simulink model "sampleModel1884_2_sub"  (R2023a)
settings: Solver=VariableStepAuto  StartTime=0.0  StopTime=10.0  RelTol=1e-3
libraries: hdlsllib x6, simulink x2
settings Model: Creator=user1  LastModifiedBy=user1

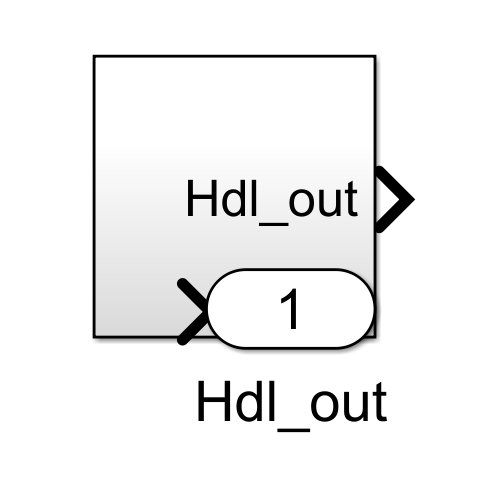
[thumbnail: Simulink's stored preview of the top-level diagram]
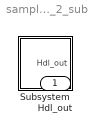
== system sampleModel1884_2_sub ==
  Subsystem : Subsystem
  Hdl_out : Outport  OutDataTypeStr=uint8

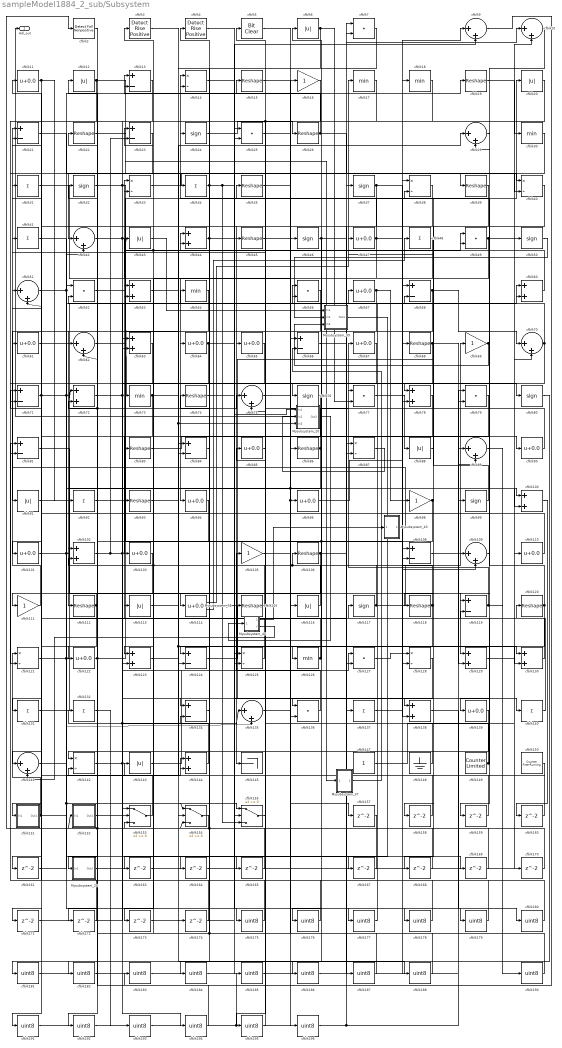
== system sampleModel1884_2_sub/Subsystem ==
  Mysubsystem_20 : Subsystem  TreatAsAtomicUnit=on  RTWFcnName=Mysubsystem_20
      settings: RTWFcnNameOpts=User specified  RTWFileNameOpts=Use function name
  Mysubsystem_28 : Subsystem  TreatAsAtomicUnit=on  RTWFcnName=Mysubsystem_28
      settings: RTWFcnNameOpts=User specified  RTWFileNameOpts=Use function name
  Mysubsystem_37 : Subsystem  TreatAsAtomicUnit=on  RTWFcnName=Mysubsystem_37
      settings: RTWFcnNameOpts=User specified  RTWFileNameOpts=Use function name
  Mysubsystem_38 : Subsystem  TreatAsAtomicUnit=on  RTWFcnName=Mysubsystem_38
      settings: RTWFcnNameOpts=User specified  RTWFileNameOpts=Use function name
  Mysubsystem_39 : Subsystem  TreatAsAtomicUnit=on  RTWFcnName=Mysubsystem_39
      settings: RTWFcnNameOpts=User specified  RTWFileNameOpts=Use function name
  Mysubsystem_40 : Subsystem  TreatAsAtomicUnit=on  RTWFcnName=Mysubsystem_40
      settings: RTWFcnNameOpts=User specified  RTWFileNameOpts=Use function name
  Mysubsystem_43 : Subsystem  TreatAsAtomicUnit=on  RTWFcnName=Mysubsystem_43
      settings: RTWFcnNameOpts=User specified  RTWFileNameOpts=Use function name
  cfblk{9..10,29,42,51,62,70,75,89,109,135,141} (12 alike) : Sum  Inputs=|++  OutDataTypeStr=uint8
  cfblk{44,53,60,63,72,78,100,102,123,129..130,138,144} (13 alike) : Sum  OutDataTypeStr=uint8
  cfblk{11,47,57,61,64..65,67,85,90,94,96,101,103,110,114,122,139} (17 alike) : Bias  Bias=0.0  SaturateOnIntegerOverflow=off
  cfblk{16,69,98,105,111} (5 alike) : Gain  OutDataTypeStr=uint8
  cfblk{15,19,22,26,35,39,45,68,74,83,86,93,106,112,115,118,120} (17 alike) : Reshape
  cfblk{13,21,23,58,66,71,81,84,108,119,124,134} (12 alike) : Sum  Inputs=+-  OutDataTypeStr=uint8
  cfblk{6,12,20,43,88,91,113,116,143} (9 alike) : Abs  OutDataTypeStr=uint8  SaturateOnIntegerOverflow=off
  cfblk{24,32,37,46,50,76,80,99,117} (9 alike) : Signum
  cfblk{14,33,38,40,87,121,125,128,142} (9 alike) : Product  Inputs=*/  OutDataTypeStr=uint8  RndMeth=Zero  SaturateOnIntegerOverflow=on
  cfblk{17..18,30,54,73,126} (6 alike) : MinMax  OutDataTypeStr=uint8
  cfblk{7,25,49,52,56,77,79,127,136} (9 alike) : DotProduct  OutDataTypeStr=uint8
  cfblk{31,34,41,48,92,131..132,137,140} (9 alike) : Sum  Inputs=+  OutDataTypeStr=uint8
  cfblk145 : Terminator
  cfblk147 : Constant  OutDataTypeStr=uint8  SampleTime=-1
  cfblk148 : Ground
  cfblk149 : hdlsllib/Sources/Counter Limited  uplimit=7  tsamp=-1
  cfblk150 : hdlsllib/Sources/Counter Free-Running  NumBits=16  tsamp=-1
  cfblk151 : Subsystem
      settings: LibrarySourceBlock=|
      | hdlsllib/Ports &
      | Subsystems/Subsystem
  cfblk152 : Subsystem
      settings: LibrarySourceBlock=|
      | hdlsllib/Ports &
      | Subsystems/Subsystem
  cfblk153 : Switch  OutDataTypeStr=uint8  SaturateOnIntegerOverflow=off  InputSameDT=off
  cfblk154 : Switch  OutDataTypeStr=uint8  SaturateOnIntegerOverflow=off  InputSameDT=off
  cfblk155 : Switch  OutDataTypeStr=uint8  SaturateOnIntegerOverflow=off  InputSameDT=off
  cfblk{157..161,163..165,167..174} (16 alike) : Delay  SampleTime=1
  cfblk{175..188,190..196} (21 alike) : DataTypeConversion  OutDataTypeStr=uint8  SaturateOnIntegerOverflow=off  RndMeth=Floor
  cfblk2 : hdlsllib/Logic and Bit Operations/Detect Fall Nonpositive  vinit=0  OutDataTypeStr=uint8
  cfblk3 : hdlsllib/Logic and Bit Operations/Detect Rise Positive  vinit=0  OutDataTypeStr=uint8
  cfblk4 : hdlsllib/Logic and Bit Operations/Detect Rise Positive  vinit=0  OutDataTypeStr=uint8
  cfblk5 : simulink/Logic and Bit Operations/Bit Clear  iBit=0
      settings: LibrarySourceBlock=|
      | hdlsllib/Logic and Bit
      | Operations/Bit Clear
  Hdl_out : Outport  OutDataTypeStr=uint8
  wires:
  cfblk73/1 -> cfblk188/1, cfblk83/1
  cfblk29/1 -> cfblk139/1
  cfblk139/1 -> cfblk142/1
  cfblk124/1 -> cfblk17/1
  cfblk122/1 -> cfblk62/2, cfblk49/1
  cfblk111/1 -> cfblk21/1
  cfblk98/1 -> cfblk168/1, cfblk186/1, cfblk154/2
  cfblk56/1 -> cfblk91/1
  cfblk69/1 -> cfblk119/1, Mysubsystem_39/3(In3)
  cfblk49/1 -> cfblk118/1, cfblk50/1
  cfblk114/1 -> cfblk140/1
  cfblk24/1 -> cfblk26/1
  cfblk131/1 -> cfblk16/1
  cfblk112/1 -> cfblk141/1, cfblk111/1
  cfblk118/1 -> cfblk134/1, cfblk53/1, cfblk106/1
  cfblk150/1 -> cfblk142/2
  cfblk83/1 -> cfblk90/1
  cfblk39/1 -> cfblk145/1
  cfblk151/1(Out1) -> cfblk121/1, cfblk154/1, cfblk144/1
  cfblk54/1 -> cfblk112/1
  cfblk88/1 -> cfblk117/1
  cfblk53/1 -> cfblk167/1, cfblk129/2
  cfblk47/1 -> cfblk9/1, cfblk123/1, cfblk14/1
  cfblk48/1 -> cfblk94/1
  cfblk63/1 -> cfblk81/2
  cfblk31/1 -> cfblk86/1
  cfblk16/1 -> cfblk65/1, cfblk121/2
  cfblk119/1 -> cfblk170/1, cfblk67/1
  cfblk108/1 -> cfblk69/1
  cfblk17/1 -> cfblk114/1
  cfblk93/1 -> cfblk29/1, Mysubsystem_20/3(In3)
  cfblk79/1 -> cfblk138/1
  cfblk40/1 -> cfblk78/1
  cfblk121/1 -> cfblk60/2, cfblk87/1
  cfblk144/1 -> cfblk12/1
  cfblk136/1 -> cfblk105/1
  cfblk26/1 -> cfblk40/2, cfblk15/1
  cfblk89/1 -> cfblk190/1
  cfblk127/1 -> cfblk128/1
  cfblk94/1 -> cfblk122/1
  cfblk71/1 -> cfblk51/2, cfblk13/2, cfblk60/1
  cfblk130/1 -> cfblk33/1
  cfblk148/1 -> cfblk41/1
  cfblk57/1 -> cfblk98/1, cfblk115/1
  cfblk76/1 -> cfblk103/1
  cfblk81/1 -> cfblk125/1
  cfblk92/1 -> cfblk24/1
  cfblk137/1 -> cfblk109/1
  cfblk152/1(Out1) -> cfblk135/1, cfblk127/1
  cfblk10/1 -> cfblk29/2
  cfblk14/1 -> cfblk45/1
  cfblk58/1 -> cfblk93/1, cfblk70/1
  cfblk115/1 -> cfblk53/2, cfblk22/1
  cfblk126/1 -> cfblk6/1, cfblk31/1
  cfblk32/1 -> cfblk155/1, cfblk108/2
  cfblk102/1 -> cfblk23/2, cfblk155/2, cfblk58/2
  cfblk128/1 -> cfblk153/2
  cfblk155/1 -> cfblk85/1
  cfblk62/1 -> cfblk20/1
  cfblk90/1 -> cfblk56/1
  cfblk13/1 -> cfblk131/1
  cfblk42/1 -> cfblk80/1, cfblk73/1
  cfblk134/1 -> cfblk54/1
  cfblk60/1 -> cfblk33/2
  cfblk110/1 -> cfblk21/2
  cfblk46/1 -> cfblk49/2, cfblk76/1
  cfblk33/1 -> cfblk39/1
  cfblk91/1 -> cfblk75/1
  cfblk68/1 -> cfblk138/2, cfblk130/1
  cfblk12/1 -> cfblk161/1, cfblk34/1
  cfblk96/1 -> cfblk38/1
  cfblk149/1 -> cfblk119/2, cfblk14/2
  cfblk44/1 -> cfblk64/1, cfblk136/1
  cfblk113/1 -> cfblk126/1
  cfblk77/1 -> cfblk88/1
  cfblk86/1 -> cfblk13/1, cfblk102/1
  cfblk132/1 -> cfblk193/1
  cfblk30/1 -> cfblk42/1
  cfblk34/1 -> cfblk124/1, cfblk9/2, cfblk155/3
  cfblk106/1 -> cfblk172/1, cfblk10/1
  cfblk120/1 -> cfblk158/1, cfblk35/1
  cfblk51/1 -> cfblk135/2, cfblk19/1
  cfblk70/1 -> cfblk123/2, cfblk52/2
  cfblk75/1 -> cfblk100/2, cfblk130/2
  cfblk74/1 -> cfblk56/2
  cfblk78/1 -> cfblk151/1(In1)
  cfblk142/1 -> cfblk164/1, cfblk134/2
  cfblk21/1 -> cfblk40/1
  cfblk129/1 -> cfblk10/2
  cfblk154/1 -> cfblk2/1
  cfblk116/1 -> cfblk43/1, cfblk23/1
  cfblk23/1 -> cfblk71/2
  cfblk143/1 -> cfblk46/1
  cfblk45/1 -> cfblk127/2, cfblk96/1
  cfblk19/1 -> cfblk30/1
  cfblk11/1 -> cfblk92/1, cfblk101/1
  cfblk101/1 -> cfblk178/1, cfblk129/1
  cfblk61/1 -> cfblk62/1
  cfblk64/1 -> cfblk192/1, Mysubsystem_20/1(In1)
  cfblk105/1 -> cfblk116/1
  cfblk135/1 -> cfblk77/1
  cfblk153/1 -> cfblk32/1, cfblk72/1
  cfblk99/1 -> cfblk38/2
  cfblk125/1 -> cfblk113/1
  cfblk140/1 -> cfblk120/1
  cfblk52/1 -> cfblk84/2
  cfblk72/1 -> cfblk194/1, cfblk78/2
  cfblk37/1 -> cfblk87/2, cfblk109/2
  cfblk6/1 -> cfblk77/2, cfblk124/2
  cfblk147/1 -> cfblk110/1
  cfblk20/1 -> cfblk63/2
  cfblk41/1 -> cfblk100/1
  cfblk117/1 -> cfblk74/1, cfblk99/1
  cfblk84/1 -> cfblk44/1
  cfblk35/1 -> cfblk157/1
  cfblk157/1 -> cfblk153/3
  cfblk158/1 -> cfblk44/2
  cfblk109/1 -> cfblk159/1
  cfblk159/1 -> cfblk71/1
  cfblk100/1 -> cfblk160/1
  cfblk160/1 -> cfblk84/1
  cfblk161/1 -> cfblk42/2
  cfblk163/1 -> cfblk136/2
  cfblk164/1 -> cfblk70/2
  cfblk141/1 -> cfblk165/1
  cfblk165/1 -> cfblk52/1
  cfblk167/1 -> cfblk153/1
  cfblk168/1 -> cfblk108/1
  cfblk15/1 -> cfblk169/1
  cfblk169/1 -> cfblk58/1
  cfblk170/1 -> cfblk102/2
  cfblk38/1 -> cfblk171/1
  cfblk171/1 -> cfblk63/1
  cfblk172/1 -> cfblk51/1
  cfblk65/1 -> cfblk173/1
  cfblk173/1 -> cfblk125/2
  cfblk123/1 -> cfblk174/1
  cfblk174/1 -> cfblk81/1
  cfblk3/1 -> cfblk175/1
  cfblk175/1 -> cfblk11/1
  cfblk67/1 -> cfblk176/1
  cfblk176/1 -> cfblk3/1
  cfblk4/1 -> cfblk177/1
  cfblk177/1 -> cfblk57/1
  cfblk178/1 -> cfblk4/1
  cfblk25/1 -> cfblk179/1
  cfblk179/1 -> cfblk75/2
  cfblk138/1 -> cfblk180/1
  cfblk180/1 -> cfblk25/1
  cfblk80/1 -> cfblk181/1
  cfblk181/1 -> cfblk25/2
  cfblk18/1 -> cfblk182/1
  cfblk182/1 -> cfblk79/1
  cfblk9/1 -> cfblk183/1
  cfblk183/1 -> cfblk18/1
  cfblk7/1 -> cfblk184/1
  cfblk184/1 -> cfblk68/1
  cfblk185/1 -> cfblk7/1
  cfblk186/1 -> cfblk7/2
  cfblk66/1 -> cfblk187/1
  cfblk187/1 -> cfblk143/1
  cfblk188/1 -> cfblk66/1
  cfblk190/1 -> cfblk144/2, cfblk154/3, cfblk152/1(In1), cfblk72/2
  cfblk103/1 -> cfblk191/1
  cfblk191/1 -> cfblk89/1
  cfblk192/1 -> cfblk89/2
  cfblk193/1 -> cfblk185/1, cfblk37/1, cfblk79/2
  cfblk194/1 -> cfblk132/1
  cfblk85/1 -> cfblk195/1
  cfblk195/1 -> cfblk5/1
  cfblk5/1 -> cfblk196/1
  cfblk196/1 -> cfblk137/1
  cfblk87/1 -> Mysubsystem_20/2(In2)
  cfblk2/1 -> Mysubsystem_28/1(In1)
  Mysubsystem_28/1(Out1) -> cfblk128/2
  cfblk22/1 -> Mysubsystem_37/1(In1)
  Mysubsystem_37/1(Out1) -> cfblk66/2
  Mysubsystem_38/1(y) -> cfblk47/1
  Mysubsystem_38/2(Out2) -> cfblk48/1
  cfblk43/1 -> Mysubsystem_39/1(In1)
  cfblk50/1 -> Mysubsystem_39/2(In2)
  Mysubsystem_39/1(Out1) -> cfblk163/1
  Mysubsystem_20/1(Out1) -> Hdl_out/1, Mysubsystem_40/1(In1)
  Mysubsystem_40/2(Y) -> cfblk141/2
  Mysubsystem_40/1(Out1) -> Mysubsystem_43/1(In1)
  Mysubsystem_43/1(Out1) -> cfblk61/1

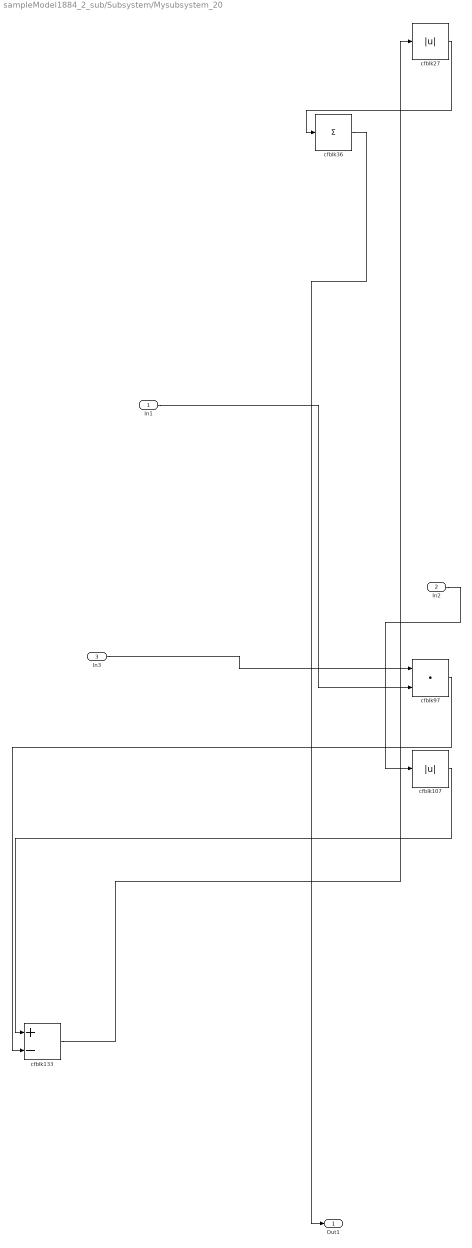
== system sampleModel1884_2_sub/Subsystem/Mysubsystem_20 ==
  In1 : Inport
  In2 : Inport  Port=2
  In3 : Inport  Port=3
  cfblk107 : Abs  SaturateOnIntegerOverflow=off
  cfblk133 : Sum  Inputs=+-
  cfblk27 : Abs  SaturateOnIntegerOverflow=off
  cfblk36 : Sum  Inputs=+
  cfblk97 : DotProduct  OutDataTypeStr=Inherit: Inherit via internal rule
  Out1 : Outport
  wires:
  In3/1 -> cfblk97/1
  In1/1 -> cfblk97/2
  cfblk107/1 -> cfblk133/1
  cfblk36/1 -> Out1/1
  cfblk27/1 -> cfblk36/1
  cfblk97/1 -> cfblk133/2
  In2/1 -> cfblk107/1
  cfblk133/1 -> cfblk27/1

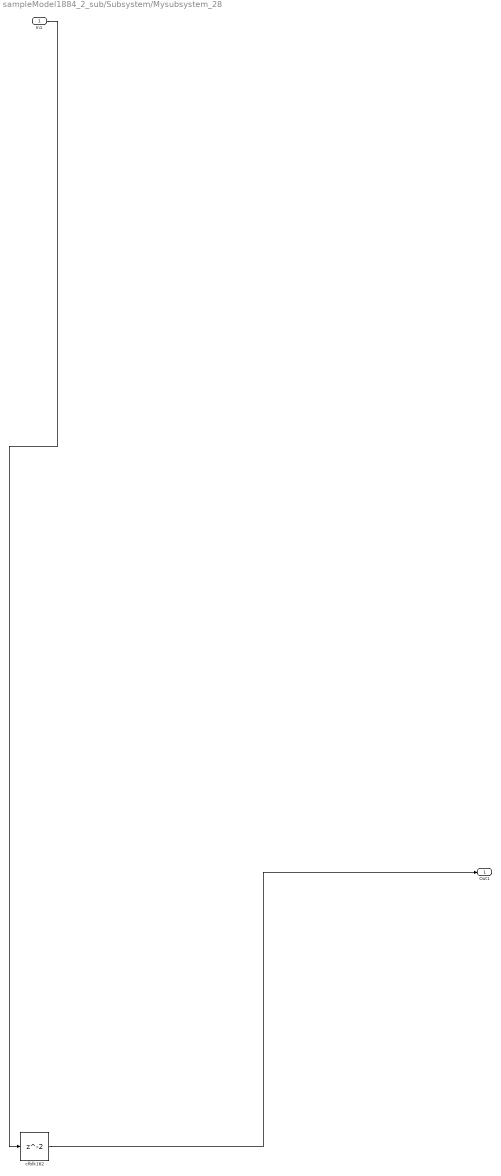
== system sampleModel1884_2_sub/Subsystem/Mysubsystem_28 ==
  In1 : Inport
  cfblk162 : Delay  SampleTime=1
  Out1 : Outport
  wires:
  In1/1 -> cfblk162/1
  cfblk162/1 -> Out1/1

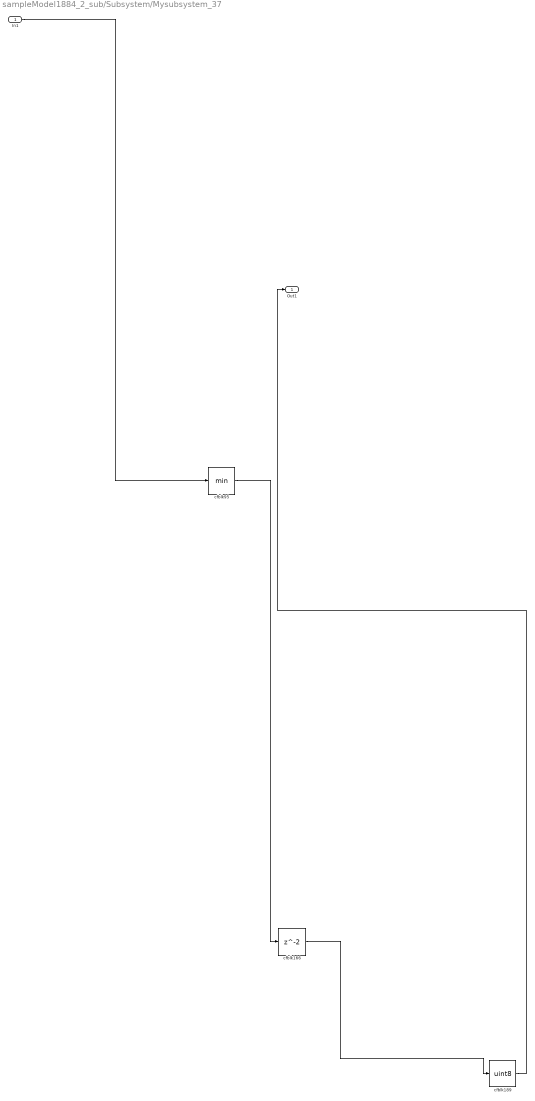
== system sampleModel1884_2_sub/Subsystem/Mysubsystem_37 ==
  In1 : Inport
  cfblk166 : Delay  SampleTime=1
  cfblk189 : DataTypeConversion  OutDataTypeStr=uint8  SaturateOnIntegerOverflow=off  RndMeth=Floor
  cfblk95 : MinMax
  Out1 : Outport
  wires:
  cfblk189/1 -> Out1/1
  In1/1 -> cfblk95/1
  cfblk95/1 -> cfblk166/1
  cfblk166/1 -> cfblk189/1

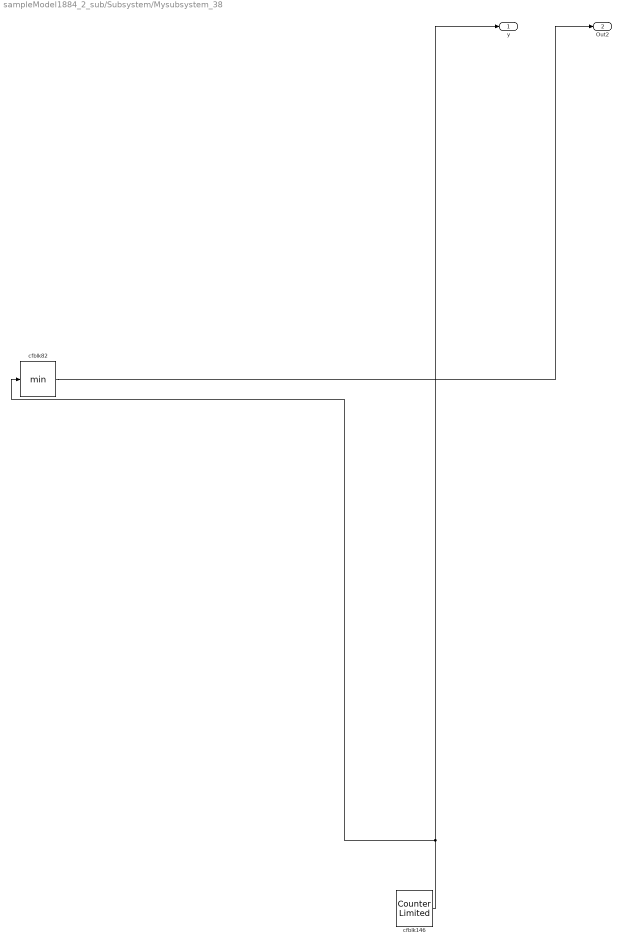
== system sampleModel1884_2_sub/Subsystem/Mysubsystem_38 ==
  cfblk146 : hdlsllib/Sources/Counter Limited  uplimit=7  tsamp=-1
  cfblk82 : MinMax
  y : Outport
  Out2 : Outport  Port=2
  wires:
  cfblk82/1 -> Out2/1
  cfblk146/1 -> cfblk82/1, y/1

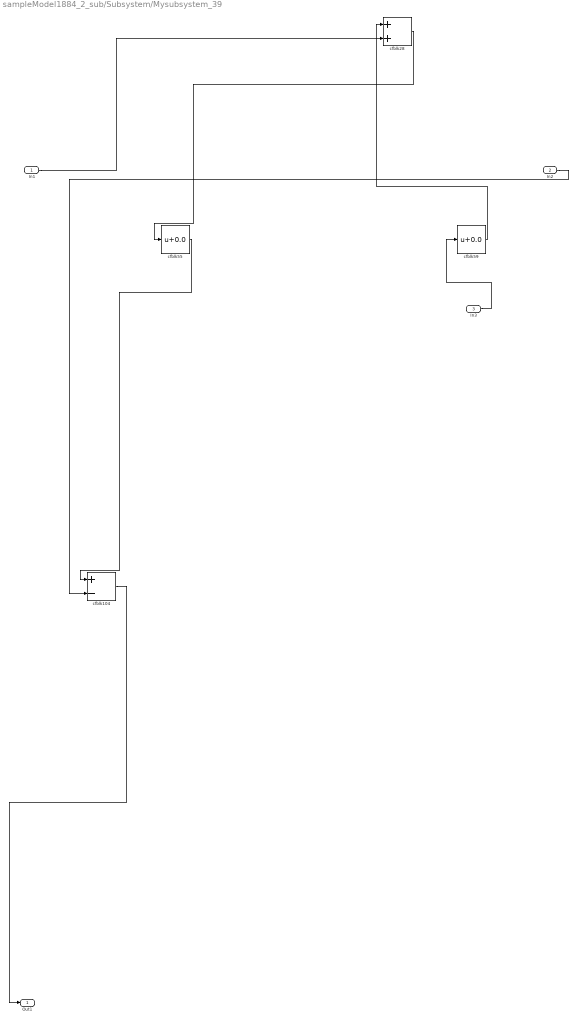
== system sampleModel1884_2_sub/Subsystem/Mysubsystem_39 ==
  In1 : Inport
  In2 : Inport  Port=2
  In3 : Inport  Port=3
  cfblk104 : Sum  Inputs=+-
  cfblk28 : Sum
  cfblk55 : Bias  Bias=0.0  SaturateOnIntegerOverflow=off
  cfblk59 : Bias  Bias=0.0  SaturateOnIntegerOverflow=off
  Out1 : Outport
  wires:
  cfblk104/1 -> Out1/1
  In2/1 -> cfblk104/2
  In3/1 -> cfblk59/1
  cfblk28/1 -> cfblk55/1
  cfblk55/1 -> cfblk104/1
  cfblk59/1 -> cfblk28/1
  In1/1 -> cfblk28/2

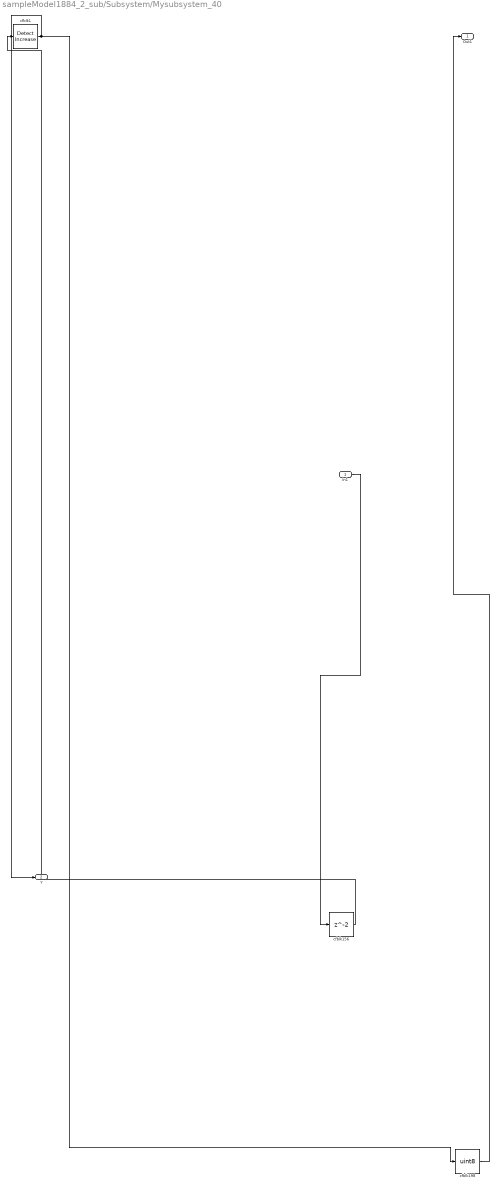
== system sampleModel1884_2_sub/Subsystem/Mysubsystem_40 ==
  In1 : Inport
  cfblk1 : simulink/Logic and Bit Operations/Detect Increase  vinit=0.0  OutDataTypeStr=boolean
      settings: LibrarySourceBlock=|
      | hdlsllib/Logic and Bit
      | Operations/Detect
      | Increase
  cfblk156 : Delay  SampleTime=1
  cfblk198 : DataTypeConversion  OutDataTypeStr=uint8  SaturateOnIntegerOverflow=off  RndMeth=Floor
  Out1 : Outport
  Y : Outport  Port=2
  wires:
  In1/1 -> cfblk156/1
  cfblk198/1 -> Out1/1
  cfblk1/1 -> cfblk198/1, Y/1
  cfblk156/1 -> cfblk1/1

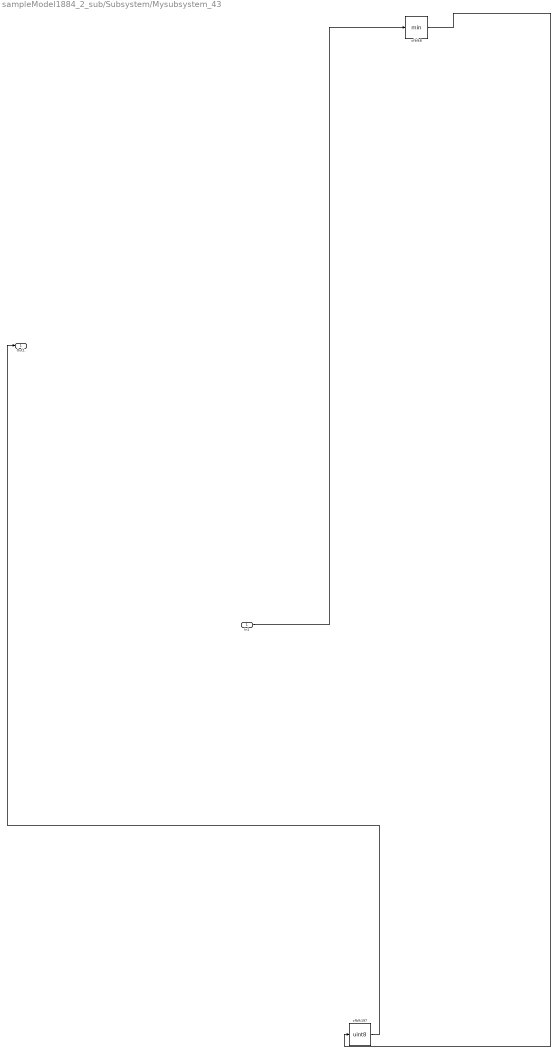
== system sampleModel1884_2_sub/Subsystem/Mysubsystem_43 ==
  In1 : Inport
  cfblk197 : DataTypeConversion  OutDataTypeStr=uint8  SaturateOnIntegerOverflow=off  RndMeth=Floor
  cfblk8 : MinMax
  Out1 : Outport
  wires:
  cfblk197/1 -> Out1/1
  In1/1 -> cfblk8/1
  cfblk8/1 -> cfblk197/1

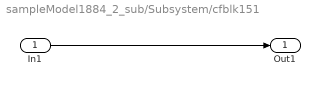
== system sampleModel1884_2_sub/Subsystem/cfblk151 ==
  In1 : Inport
  Out1 : Outport
  wires:
  In1/1 -> Out1/1

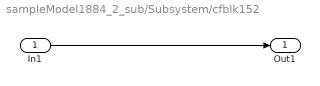
== system sampleModel1884_2_sub/Subsystem/cfblk152 ==
  In1 : Inport
  Out1 : Outport
  wires:
  In1/1 -> Out1/1
